simulink model "robotarm_part_2"  (R2018b)
settings: Solver=FixedStepAuto  StartTime=0.0  StopTime=options.T_train  RelTol=1e-3  AbsTol=1e-6
undefined symbols (not defined in the file): options
libraries: neural x132, simulink x2
(part 2 of 6)

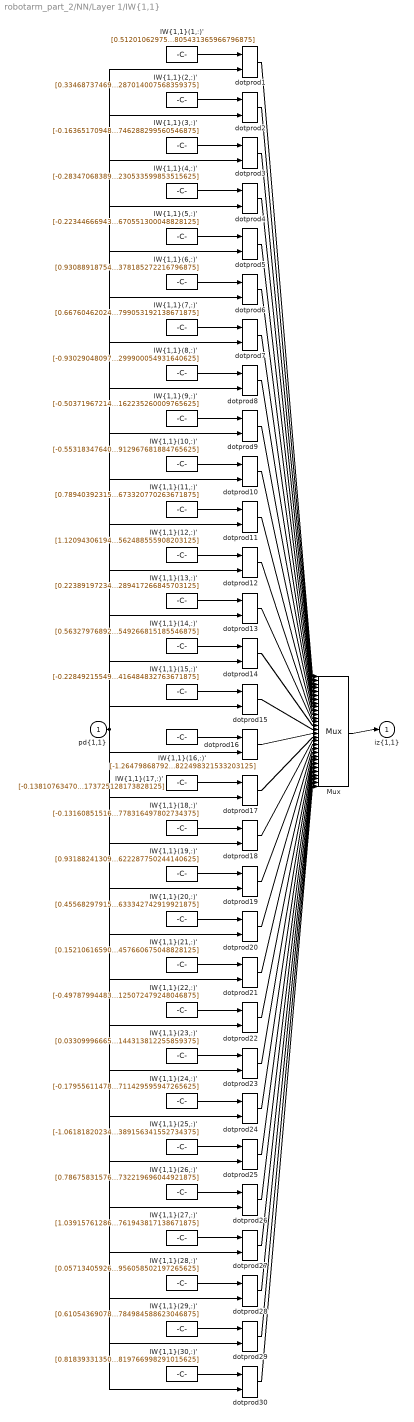
== system robotarm_part_2/NN/Layer 1/IW{1,1} ==
  "pd{1,1}" : Inport  PortDimensions=10
      mask Display: e = 0.06;c1 = [120 230 180]/255;c2 = ([120 230 180]+0)/(256+128);c3 = ([120 230 180]+128)/(256+128);patch([0 1 1 0],[0 0 1 1],c1);patch([0 1 1 1-e 1-e 0+e],[0 0 1 1-e 0+e 0+e],c2);patch([0 0 1 1-e 0+e 0+e],[0 1 1 1-e 1-e 0+e],c3);plot([0 1 1 0 0],[0 0 1 1 0]);
  "IW{1,1}(1,:)'" : Constant  Value=[0.51201062975041689018240731456899084150791168212890625;-0.446218385660316740892739062473992817103862762451171875;-0.82313455567312721061767888386384584009647369384765625;0.67500458565279519707047484189388342201709747314453125;-1.0822077647345456075100855741766281425952911376953125;0.744755827537209480482260914868675172328948974609375;0.61245740151635452708234197416459210216999053955078125;-0.411857215597841774812337689581909216940402984619140625;-0.060313846036639418013436397814075462520122528076171875;0.149541145773167016841398435644805431365966796875]
      mask Display: e = 0.06;c1 = [120 150 230]/255;c2 = ([120 150 230]+0)/383;c3 = ([120 150 230]+128)/383;patch([0 1 1 0],[0 0 1 1],c1);patch([0 1 1 1-e 1-e 0+e],[0 0 1 1-e 0+e 0+e],c2);patch([0 0 1 1-e 0+e 0+e],[0 1 1 1-e 1-e 0+e],c3);plot([0 1 1 0 0],[0 0 1 1 0]);disp('Weights');
  "IW{1,1}(10,:)'" : Constant  Value=[-0.5531834764078296107214782750816084444522857666015625;0.84193722423272554511441967406426556408405303955078125;-0.2314244047025942052631108936111559160053730010986328125;1.268304889703578464121846991474740207195281982421875;-0.298486853726749934434536726257647387683391571044921875;-0.58903786713781192130312547305948100984096527099609375;-0.144387121841211774064817063845111988484859466552734375;1.0323527503820091322239704823005013167858123779296875;-0.5268015142183148924459601403214037418365478515625;-0.294966032842409353609269828666583634912967681884765625]
      mask Display: e = 0.06;c1 = [120 150 230]/255;c2 = ([120 150 230]+0)/383;c3 = ([120 150 230]+128)/383;patch([0 1 1 0],[0 0 1 1],c1);patch([0 1 1 1-e 1-e 0+e],[0 0 1 1-e 0+e 0+e],c2);patch([0 0 1 1-e 0+e 0+e],[0 1 1 1-e 1-e 0+e],c3);plot([0 1 1 0 0],[0 0 1 1 0]);disp('Weights');
  "IW{1,1}(11,:)'" : Constant  Value=[0.78940392315049578986219103171606548130512237548828125;-0.59945395218989439012347020252491347491741180419921875;0.301682263197468436555226389828021638095378875732421875;0.250976303480782869659293510267161764204502105712890625;-0.270480787649907572500751484767533838748931884765625;-0.804027705366989753343887059600092470645904541015625;1.2521368901740081991391662086243741214275360107421875;0.657348093834792646106279789819382131099700927734375;-0.146075233696211059797320785946794785559177398681640625;-0.1885013219685194030272867848907480947673320770263671875]
      mask Display: e = 0.06;c1 = [120 150 230]/255;c2 = ([120 150 230]+0)/383;c3 = ([120 150 230]+128)/383;patch([0 1 1 0],[0 0 1 1],c1);patch([0 1 1 1-e 1-e 0+e],[0 0 1 1-e 0+e 0+e],c2);patch([0 0 1 1-e 0+e 0+e],[0 1 1 1-e 1-e 0+e],c3);plot([0 1 1 0 0],[0 0 1 1 0]);disp('Weights');
  "IW{1,1}(12,:)'" : Constant  Value=[1.120943061943604934782570126117207109928131103515625;-0.1777527950664744837983022307525970973074436187744140625;1.1402714559446653908025837154127657413482666015625;1.6329959194421557189258464859449304640293121337890625;1.799945318979037978124324581585824489593505859375;0.8358067878004415973691720864735543727874755859375;1.064775855755599298646529859979636967182159423828125;-0.152682851516850404127723095371038652956485748291015625;-0.96941769778080966180056066150427795946598052978515625;-0.644809351839978450726675873738713562488555908203125]
      mask Display: e = 0.06;c1 = [120 150 230]/255;c2 = ([120 150 230]+0)/383;c3 = ([120 150 230]+128)/383;patch([0 1 1 0],[0 0 1 1],c1);patch([0 1 1 1-e 1-e 0+e],[0 0 1 1-e 0+e 0+e],c2);patch([0 0 1 1-e 0+e 0+e],[0 1 1 1-e 1-e 0+e],c3);plot([0 1 1 0 0],[0 0 1 1 0]);disp('Weights');
  "IW{1,1}(13,:)'" : Constant  Value=[0.2238919723487180213350455915133352391421794891357421875;0.597710842623245586224811631836928427219390869140625;-0.055930922318855595676279079953019390814006328582763671875;0.97815912828886653063165113053401000797748565673828125;-0.5914319335257880450029688290669582784175872802734375;-0.595428981931443335184894749545492231845855712890625;0.0681264786780833853097050223368569277226924896240234375;1.1822948963348218764934927094145677983760833740234375;0.014091328986622152219521098004406667314469814300537109375;-0.232872425589578935234413847865653224289417266845703125]
      mask Display: e = 0.06;c1 = [120 150 230]/255;c2 = ([120 150 230]+0)/383;c3 = ([120 150 230]+128)/383;patch([0 1 1 0],[0 0 1 1],c1);patch([0 1 1 1-e 1-e 0+e],[0 0 1 1-e 0+e 0+e],c2);patch([0 0 1 1-e 0+e 0+e],[0 1 1 1-e 1-e 0+e],c3);plot([0 1 1 0 0],[0 0 1 1 0]);disp('Weights');
  "IW{1,1}(14,:)'" : Constant  Value=[0.56327976892860409652286080017802305519580841064453125;-0.83851149677898872969450394521118141710758209228515625;0.3782787095400166332836988658527843654155731201171875;-0.2423293037754235268455005325449747033417224884033203125;-0.60723210282409489924049239562009461224079132080078125;1.3496313158650192765009023787570185959339141845703125;-1.068818057232499452169349751784466207027435302734375;0.428137373095577367099195953414891846477985382080078125;0.70485126250453256080419350837473757565021514892578125;-0.304558790502350074103077304243925027549266815185546875]
      mask Display: e = 0.06;c1 = [120 150 230]/255;c2 = ([120 150 230]+0)/383;c3 = ([120 150 230]+128)/383;patch([0 1 1 0],[0 0 1 1],c1);patch([0 1 1 1-e 1-e 0+e],[0 0 1 1-e 0+e 0+e],c2);patch([0 0 1 1-e 0+e 0+e],[0 1 1 1-e 1-e 0+e],c3);plot([0 1 1 0 0],[0 0 1 1 0]);disp('Weights');
  "IW{1,1}(15,:)'" : Constant  Value=[-0.2284921554935588627888165547119569964706897735595703125;1.3167348428603504739697882541804574429988861083984375;-1.183745976367202690227031780523248016834259033203125;0.3104414845865590688589463752578012645244598388671875;-0.24879563196083387399681896567926742136478424072265625;-0.8014990752859769695959357704850845038890838623046875;0.97682041688133935952720321438391692936420440673828125;0.9148661125020822737496928311884403228759765625;-0.53839922957077013254689745735959149897098541259765625;0.0629641058630556471609196478311787359416484832763671875]
      mask Display: e = 0.06;c1 = [120 150 230]/255;c2 = ([120 150 230]+0)/383;c3 = ([120 150 230]+128)/383;patch([0 1 1 0],[0 0 1 1],c1);patch([0 1 1 1-e 1-e 0+e],[0 0 1 1-e 0+e 0+e],c2);patch([0 0 1 1-e 0+e 0+e],[0 1 1 1-e 1-e 0+e],c3);plot([0 1 1 0 0],[0 0 1 1 0]);disp('Weights');
  "IW{1,1}(16,:)'" : Constant  Value=[-1.264798687929534093399297489668242633342742919921875;-0.8666288950522902378992284866399131715297698974609375;-0.351867621039619382639074274266022257506847381591796875;-1.2235468539213540939414315289468504488468170166015625;-0.69647725102835267296796928349067457020282745361328125;-0.336143791072206876702210820440086536109447479248046875;-2.07998144178045407670651911757886409759521484375;0.42152524350633291394530033358023501932621002197265625;-0.54013888040281232694184154752292670309543609619140625;0.27962398287528611451335791571182198822498321533203125]
      mask Display: e = 0.06;c1 = [120 150 230]/255;c2 = ([120 150 230]+0)/383;c3 = ([120 150 230]+128)/383;patch([0 1 1 0],[0 0 1 1],c1);patch([0 1 1 1-e 1-e 0+e],[0 0 1 1-e 0+e 0+e],c2);patch([0 0 1 1-e 0+e 0+e],[0 1 1 1-e 1-e 0+e],c3);plot([0 1 1 0 0],[0 0 1 1 0]);disp('Weights');
  "IW{1,1}(17,:)'" : Constant  Value=[-0.138107634700562698082393353615771047770977020263671875;-0.6829199452269809622606544508016668260097503662109375;0.1872812962193503294461294217398972250521183013916015625;0.996618728469853554230439840466715395450592041015625;0.70601568915720169794525418183184228837490081787109375;0.71409007827887716057801981150987558066844940185546875;-0.05393398252795689185035143964341841638088226318359375;0.54491065742438049568363567232154309749603271484375;0.71411317961737508230868343162001110613346099853515625;-0.1686958312051092534478158313504536636173725128173828125]
      mask Display: e = 0.06;c1 = [120 150 230]/255;c2 = ([120 150 230]+0)/383;c3 = ([120 150 230]+128)/383;patch([0 1 1 0],[0 0 1 1],c1);patch([0 1 1 1-e 1-e 0+e],[0 0 1 1-e 0+e 0+e],c2);patch([0 0 1 1-e 0+e 0+e],[0 1 1 1-e 1-e 0+e],c3);plot([0 1 1 0 0],[0 0 1 1 0]);disp('Weights');
  "IW{1,1}(18,:)'" : Constant  Value=[-0.1316085151623478111115872479786048643290996551513671875;0.1705613878097677893475037080861511640250682830810546875;-0.0962470582835133203758459785603918135166168212890625;-0.91249714780919777279422078208881430327892303466796875;-1.158643775472975701035238671465776860713958740234375;0.068576612657344160339789596037007868289947509765625;0.35933323325870480946520046927616931498050689697265625;0.93664609339309568003528738699969835579395294189453125;0.6175964938953411031974383149645291268825531005859375;0.53882994034340947475669736377312801778316497802734375]
      mask Display: e = 0.06;c1 = [120 150 230]/255;c2 = ([120 150 230]+0)/383;c3 = ([120 150 230]+128)/383;patch([0 1 1 0],[0 0 1 1],c1);patch([0 1 1 1-e 1-e 0+e],[0 0 1 1-e 0+e 0+e],c2);patch([0 0 1 1-e 0+e 0+e],[0 1 1 1-e 1-e 0+e],c3);plot([0 1 1 0 0],[0 0 1 1 0]);disp('Weights');
  "IW{1,1}(19,:)'" : Constant  Value=[0.93188241309977526416474802317679859697818756103515625;0.3431987483161054175440085600712336599826812744140625;0.8149782526990210218542642905958928167819976806640625;-0.48223366783551668834917336425860412418842315673828125;-1.2205060054262257818180614776792936027050018310546875;-0.518485301399788767184872995130717754364013671875;0.1822236035677796961440577661051065661013126373291015625;0.59438057885021955417670369570259936153888702392578125;0.290405258873669025465602544500143267214298248291015625;-0.227514175994425971172319123070337809622287750244140625]
      mask Display: e = 0.06;c1 = [120 150 230]/255;c2 = ([120 150 230]+0)/383;c3 = ([120 150 230]+128)/383;patch([0 1 1 0],[0 0 1 1],c1);patch([0 1 1 1-e 1-e 0+e],[0 0 1 1-e 0+e 0+e],c2);patch([0 0 1 1-e 0+e 0+e],[0 1 1 1-e 1-e 0+e],c3);plot([0 1 1 0 0],[0 0 1 1 0]);disp('Weights');
  "IW{1,1}(2,:)'" : Constant  Value=[0.334687374696120254480291578147443942725658416748046875;0.8542580739553733426561166197643615305423736572265625;-0.300144445451211716591188860547845251858234405517578125;0.208731003203754206243303315204684622585773468017578125;-0.85850869408691499184982376391417346894741058349609375;-0.8662264510329513722552974286372773349285125732421875;0.22452379060819982470320610445924103260040283203125;0.15532066551018408606665843763039447367191314697265625;0.1101313638464642696845885438960976898670196533203125;-0.869876084554048301100692697218619287014007568359375]
      mask Display: e = 0.06;c1 = [120 150 230]/255;c2 = ([120 150 230]+0)/383;c3 = ([120 150 230]+128)/383;patch([0 1 1 0],[0 0 1 1],c1);patch([0 1 1 1-e 1-e 0+e],[0 0 1 1-e 0+e 0+e],c2);patch([0 0 1 1-e 0+e 0+e],[0 1 1 1-e 1-e 0+e],c3);plot([0 1 1 0 0],[0 0 1 1 0]);disp('Weights');
  "IW{1,1}(20,:)'" : Constant  Value=[0.455682979150963729519929756861529313027858734130859375;-0.348772677236663664057658706951770000159740447998046875;-1.081291878654035532036914446507580578327178955078125;0.6215181655236268198905236204154789447784423828125;-1.26078388760682447156113994424231350421905517578125;0.26210421145090878614070106777944602072238922119140625;-0.8124006863890798069149923321674577891826629638671875;-0.7488565667669575542930715528200380504131317138671875;-0.022788057892801479031863465252172318287193775177001953125;-0.569162418060251251716863407636992633342742919921875]
      mask Display: e = 0.06;c1 = [120 150 230]/255;c2 = ([120 150 230]+0)/383;c3 = ([120 150 230]+128)/383;patch([0 1 1 0],[0 0 1 1],c1);patch([0 1 1 1-e 1-e 0+e],[0 0 1 1-e 0+e 0+e],c2);patch([0 0 1 1-e 0+e 0+e],[0 1 1 1-e 1-e 0+e],c3);plot([0 1 1 0 0],[0 0 1 1 0]);disp('Weights');
  "IW{1,1}(21,:)'" : Constant  Value=[0.15210616590676995230069223907776176929473876953125;-0.52353059267904367146684307954274117946624755859375;-0.06401275842094468482290636757170432247221469879150390625;0.8786379509407431509515618017758242785930633544921875;-0.984808213135992094322546108742244541645050048828125;-0.80881132688778212269653522525914013385772705078125;1.0254205955323396626255316732567735016345977783203125;-0.572903581729212962869723924086429178714752197265625;-0.57828165266377162812005963132833130657672882080078125;-0.0981817788360586363172188839598675258457660675048828125]
      mask Display: e = 0.06;c1 = [120 150 230]/255;c2 = ([120 150 230]+0)/383;c3 = ([120 150 230]+128)/383;patch([0 1 1 0],[0 0 1 1],c1);patch([0 1 1 1-e 1-e 0+e],[0 0 1 1-e 0+e 0+e],c2);patch([0 0 1 1-e 0+e 0+e],[0 1 1 1-e 1-e 0+e],c3);plot([0 1 1 0 0],[0 0 1 1 0]);disp('Weights');
  "IW{1,1}(22,:)'" : Constant  Value=[-0.49787994483490027874950101249851286411285400390625;0.344426173820214842624665152470697648823261260986328125;0.56655019007916529449886411384795792400836944580078125;-0.1743990939602932666030454811334493570029735565185546875;-0.55634090371249012019205792967113666236400604248046875;0.89898279581140183580600933055393397808074951171875;-0.879074509234978318517050865921191871166229248046875;0.35855501727174743376025389807182364165782928466796875;-0.35938092675222998995110401665442623198032379150390625;0.259808285173537878431915260080131702125072479248046875]
      mask Display: e = 0.06;c1 = [120 150 230]/255;c2 = ([120 150 230]+0)/383;c3 = ([120 150 230]+128)/383;patch([0 1 1 0],[0 0 1 1],c1);patch([0 1 1 1-e 1-e 0+e],[0 0 1 1-e 0+e 0+e],c2);patch([0 0 1 1-e 0+e 0+e],[0 1 1 1-e 1-e 0+e],c3);plot([0 1 1 0 0],[0 0 1 1 0]);disp('Weights');
  "IW{1,1}(23,:)'" : Constant  Value=[0.033099966659816792979853516953880898654460906982421875;0.06638646623711309813220537989764125086367130279541015625;-0.68962437461610448519166993719409219920635223388671875;-0.7036292898254934424784323709900490939617156982421875;1.2199498264654824453145920415408909320831298828125;-0.79167659947821267252265897695906460285186767578125;-0.77727190827501690950640522714820690453052520751953125;-0.86932059827218122194381066947244107723236083984375;-1.30799569035398377536694169975817203521728515625;0.61475854294593756943498874534270726144313812255859375]
      mask Display: e = 0.06;c1 = [120 150 230]/255;c2 = ([120 150 230]+0)/383;c3 = ([120 150 230]+128)/383;patch([0 1 1 0],[0 0 1 1],c1);patch([0 1 1 1-e 1-e 0+e],[0 0 1 1-e 0+e 0+e],c2);patch([0 0 1 1-e 0+e 0+e],[0 1 1 1-e 1-e 0+e],c3);plot([0 1 1 0 0],[0 0 1 1 0]);disp('Weights');
  "IW{1,1}(24,:)'" : Constant  Value=[-0.179556114788564202822129800551920197904109954833984375;-1.087956549232024006101937629864551126956939697265625;-0.491519599031757403739817391397082246840000152587890625;0.431654739378498575330667108573834411799907684326171875;-0.5203235292342416329347543069161474704742431640625;1.0774856436627977540609890638734214007854461669921875;-0.78412901417916491819681823471910320222377777099609375;-0.45999524609127895313775979957426898181438446044921875;-0.65676880719675245767774640626157633960247039794921875;-0.044675480221918285883564436744563863612711429595947265625]
      mask Display: e = 0.06;c1 = [120 150 230]/255;c2 = ([120 150 230]+0)/383;c3 = ([120 150 230]+128)/383;patch([0 1 1 0],[0 0 1 1],c1);patch([0 1 1 1-e 1-e 0+e],[0 0 1 1-e 0+e 0+e],c2);patch([0 0 1 1-e 0+e 0+e],[0 1 1 1-e 1-e 0+e],c3);plot([0 1 1 0 0],[0 0 1 1 0]);disp('Weights');
  "IW{1,1}(25,:)'" : Constant  Value=[-1.0618182023466058438998516066931188106536865234375;0.79817916296788327112921024308889172971248626708984375;0.66539862575941655098432647719164378941059112548828125;-0.051018015239275439631772002258003340102732181549072265625;-1.0134808839080953202227419751579873263835906982421875;0.32366586780373907128449673109571449458599090576171875;-0.77640544809128508862983153449022211134433746337890625;0.052087738911195731461578617427221615798771381378173828125;0.356415790452184799708135187756852246820926666259765625;-0.82901405933345040377702162004425190389156341552734375]
      mask Display: e = 0.06;c1 = [120 150 230]/255;c2 = ([120 150 230]+0)/383;c3 = ([120 150 230]+128)/383;patch([0 1 1 0],[0 0 1 1],c1);patch([0 1 1 1-e 1-e 0+e],[0 0 1 1-e 0+e 0+e],c2);patch([0 0 1 1-e 0+e 0+e],[0 1 1 1-e 1-e 0+e],c3);plot([0 1 1 0 0],[0 0 1 1 0]);disp('Weights');
  "IW{1,1}(26,:)'" : Constant  Value=[0.7867583157629229884122423754888586699962615966796875;-0.09876131895016322659319740751016070134937763214111328125;0.040937343456810305897253243756495066918432712554931640625;-0.6377087573054336377964546045404858887195587158203125;0.92183111098579606501601801937795244157314300537109375;0.7630701117262292942911017235019244253635406494140625;-0.9559463989704750641607233774266205728054046630859375;0.0083999903600966881189737733848232892341911792755126953125;0.28071027682913085588012336302199400961399078369140625;-0.356962075893640651269578256687964312732219696044921875]
      mask Display: e = 0.06;c1 = [120 150 230]/255;c2 = ([120 150 230]+0)/383;c3 = ([120 150 230]+128)/383;patch([0 1 1 0],[0 0 1 1],c1);patch([0 1 1 1-e 1-e 0+e],[0 0 1 1-e 0+e 0+e],c2);patch([0 0 1 1-e 0+e 0+e],[0 1 1 1-e 1-e 0+e],c3);plot([0 1 1 0 0],[0 0 1 1 0]);disp('Weights');
  "IW{1,1}(27,:)'" : Constant  Value=[1.0391576128606516693508865500916726887226104736328125;-0.68078374226108329114737216514186002314090728759765625;-0.84542657228553519388469794648699462413787841796875;0.182872090681562127212345103544066660106182098388671875;0.201449348403338335256052005206583999097347259521484375;1.2222722009825515154801678363583050668239593505859375;-0.209857643206624533416260192097979597747325897216796875;-0.0260964357222159791527271721633951528929173946380615234375;0.032308480457565631749350387735830736346542835235595703125;-0.32241355661655546338550948348711244761943817138671875]
      mask Display: e = 0.06;c1 = [120 150 230]/255;c2 = ([120 150 230]+0)/383;c3 = ([120 150 230]+128)/383;patch([0 1 1 0],[0 0 1 1],c1);patch([0 1 1 1-e 1-e 0+e],[0 0 1 1-e 0+e 0+e],c2);patch([0 0 1 1-e 0+e 0+e],[0 1 1 1-e 1-e 0+e],c3);plot([0 1 1 0 0],[0 0 1 1 0]);disp('Weights');
  "IW{1,1}(28,:)'" : Constant  Value=[0.057134059266083149497550408568713464774191379547119140625;0.9612957029473683245868187441374175250530242919921875;-0.82745424130805333984284288817434571683406829833984375;-0.358522123753254928768541276440373621881008148193359375;-0.370650427652782610277171215784619562327861785888671875;0.79355103244975133680583212480996735394001007080078125;-0.585900745193040695113495530677028000354766845703125;-0.3012560077043449080491654967772774398326873779296875;-0.59586095918726922349151209346018731594085693359375;0.06521372026171236291336441581734106875956058502197265625]
      mask Display: e = 0.06;c1 = [120 150 230]/255;c2 = ([120 150 230]+0)/383;c3 = ([120 150 230]+128)/383;patch([0 1 1 0],[0 0 1 1],c1);patch([0 1 1 1-e 1-e 0+e],[0 0 1 1-e 0+e 0+e],c2);patch([0 0 1 1-e 0+e 0+e],[0 1 1 1-e 1-e 0+e],c3);plot([0 1 1 0 0],[0 0 1 1 0]);disp('Weights');
  "IW{1,1}(29,:)'" : Constant  Value=[0.61054369078136849768867477905587293207645416259765625;0.285441813611004846507057663984596729278564453125;0.82694574023073530444349898971267975866794586181640625;-0.95255589439435184306859127900679595768451690673828125;-0.7232895052037340288819677880383096635341644287109375;0.052786005032112760793072681053672567941248416900634765625;0.32963064971604894015655418115784414112567901611328125;-0.361308139964405972133221212061471305787563323974609375;-0.0607358777905373237171460232275421731173992156982421875;0.365889917645603357509997977103921584784984588623046875]
      mask Display: e = 0.06;c1 = [120 150 230]/255;c2 = ([120 150 230]+0)/383;c3 = ([120 150 230]+128)/383;patch([0 1 1 0],[0 0 1 1],c1);patch([0 1 1 1-e 1-e 0+e],[0 0 1 1-e 0+e 0+e],c2);patch([0 0 1 1-e 0+e 0+e],[0 1 1 1-e 1-e 0+e],c3);plot([0 1 1 0 0],[0 0 1 1 0]);disp('Weights');
  "IW{1,1}(3,:)'" : Constant  Value=[-0.1636517094816495043740900428019813261926174163818359375;0.2790709887831928082135846125311218202114105224609375;-0.82095080725694657974855772408773191273212432861328125;0.90315988282876080717187505797483026981353759765625;-0.585383166098789597953100383165292441844940185546875;-0.9028020381220780432585115704569034278392791748046875;-0.55194084143176491696891616811626590788364410400390625;-0.80841281361235195479508774951682426035404205322265625;-0.1330243909813022262778048343534464947879314422607421875;-0.79353581713547594045365940473857335746288299560546875]
      mask Display: e = 0.06;c1 = [120 150 230]/255;c2 = ([120 150 230]+0)/383;c3 = ([120 150 230]+128)/383;patch([0 1 1 0],[0 0 1 1],c1);patch([0 1 1 1-e 1-e 0+e],[0 0 1 1-e 0+e 0+e],c2);patch([0 0 1 1-e 0+e 0+e],[0 1 1 1-e 1-e 0+e],c3);plot([0 1 1 0 0],[0 0 1 1 0]);disp('Weights');
  "IW{1,1}(30,:)'" : Constant  Value=[0.81839331350390442931796997072524391114711761474609375;-0.65665848396522774610417627627612091600894927978515625;-0.62904998603653716759964709126506932079792022705078125;-0.244816186549569547725724305564654059708118438720703125;0.7943841339580812732634740314097143709659576416015625;0.9540530841623862112754750341991893947124481201171875;0.222742363091552320053523317255894653499126434326171875;-0.40821844777976334928126789236557669937610626220703125;-0.5056520505561186151766150942421518266201019287109375;0.5224344282092714397691679550916887819766998291015625]
      mask Display: e = 0.06;c1 = [120 150 230]/255;c2 = ([120 150 230]+0)/383;c3 = ([120 150 230]+128)/383;patch([0 1 1 0],[0 0 1 1],c1);patch([0 1 1 1-e 1-e 0+e],[0 0 1 1-e 0+e 0+e],c2);patch([0 0 1 1-e 0+e 0+e],[0 1 1 1-e 1-e 0+e],c3);plot([0 1 1 0 0],[0 0 1 1 0]);disp('Weights');
  "IW{1,1}(4,:)'" : Constant  Value=[-0.283470683898927433563841304930974729359149932861328125;-0.566705526229471789889657884486950933933258056640625;-0.0683239219797149299751026774174533784389495849609375;-0.334143830811465314400976467368309386074542999267578125;-0.7385101067126182972089054601383395493030548095703125;0.085369537996802635770876577225863002240657806396484375;0.508384686137323793531095361686311662197113037109375;1.3096152971670582676466665361658670008182525634765625;-0.80825421096264238318696015994646586477756500244140625;-0.73138548990404628202810499715269543230533599853515625]
      mask Display: e = 0.06;c1 = [120 150 230]/255;c2 = ([120 150 230]+0)/383;c3 = ([120 150 230]+128)/383;patch([0 1 1 0],[0 0 1 1],c1);patch([0 1 1 1-e 1-e 0+e],[0 0 1 1-e 0+e 0+e],c2);patch([0 0 1 1-e 0+e 0+e],[0 1 1 1-e 1-e 0+e],c3);plot([0 1 1 0 0],[0 0 1 1 0]);disp('Weights');
  "IW{1,1}(5,:)'" : Constant  Value=[-0.22344666943307378570438004317111335694789886474609375;0.55446481881344722442150896313250996172428131103515625;-0.6986360943472436080270426828064955770969390869140625;0.1859580900224321042824016103622852824628353118896484375;-0.67870494890880450622461239618132822215557098388671875;-0.586692796095814816936808711034245789051055908203125;0.09071355422038583637966979722477844916284084320068359375;0.25741529128786100333314834642806090414524078369140625;-0.77523298959876674185665024197078309953212738037109375;-0.3024283743969693460940106888301670551300048828125]
      mask Display: e = 0.06;c1 = [120 150 230]/255;c2 = ([120 150 230]+0)/383;c3 = ([120 150 230]+128)/383;patch([0 1 1 0],[0 0 1 1],c1);patch([0 1 1 1-e 1-e 0+e],[0 0 1 1-e 0+e 0+e],c2);patch([0 0 1 1-e 0+e 0+e],[0 1 1 1-e 1-e 0+e],c3);plot([0 1 1 0 0],[0 0 1 1 0]);disp('Weights');
  "IW{1,1}(6,:)'" : Constant  Value=[0.9308891875477172117570034970412962138652801513671875;0.6248987167310067203374046584940515458583831787109375;-0.421406323878703081842189703820622526109218597412109375;-0.5088996357030708406199437376926653087139129638671875;-0.8857877018437314564636153590981848537921905517578125;-0.2069905306570896386109126297014881856739521026611328125;-1.0089923907319573448404526061494834721088409423828125;0.08415741437822508996813297699191025458276271820068359375;0.97591180294049617582885502997669391334056854248046875;-0.388183431962278557847412230330519378185272216796875]
      mask Display: e = 0.06;c1 = [120 150 230]/255;c2 = ([120 150 230]+0)/383;c3 = ([120 150 230]+128)/383;patch([0 1 1 0],[0 0 1 1],c1);patch([0 1 1 1-e 1-e 0+e],[0 0 1 1-e 0+e 0+e],c2);patch([0 0 1 1-e 0+e 0+e],[0 1 1 1-e 1-e 0+e],c3);plot([0 1 1 0 0],[0 0 1 1 0]);disp('Weights');
  "IW{1,1}(7,:)'" : Constant  Value=[0.66760462024022715343818390465457923710346221923828125;-0.333285831523196518499929652534774504601955413818359375;0.0154658587186106109834238253597504808567464351654052734375;0.015814647545966863118049872127812705002725124359130859375;-0.81793240186973459326935653734835796058177947998046875;-0.33959407024115029205546534285531379282474517822265625;-1.5662660277990558821414879275835119187831878662109375;-0.87198956266450411423107880182215012609958648681640625;0.351466567986612410390279137573088519275188446044921875;0.398619991678556828684776291993330232799053192138671875]
      mask Display: e = 0.06;c1 = [120 150 230]/255;c2 = ([120 150 230]+0)/383;c3 = ([120 150 230]+128)/383;patch([0 1 1 0],[0 0 1 1],c1);patch([0 1 1 1-e 1-e 0+e],[0 0 1 1-e 0+e 0+e],c2);patch([0 0 1 1-e 0+e 0+e],[0 1 1 1-e 1-e 0+e],c3);plot([0 1 1 0 0],[0 0 1 1 0]);disp('Weights');
  "IW{1,1}(8,:)'" : Constant  Value=[-0.9302904809764058757792781761963851749897003173828125;0.45922692721911317903504823334515094757080078125;-0.95093316525850790643659138368093408644199371337890625;-0.93733031649115894357038314410601742565631866455078125;-0.10339789326997579632649859604498487897217273712158203125;0.476935800121459585465544250837410800158977508544921875;0.47368795097230564916657158391899429261684417724609375;0.149512630423817183267232167054316960275173187255859375;-0.87451657742440003229233980164281092584133148193359375;-0.06311678743072259012425462287865229882299900054931640625]
      mask Display: e = 0.06;c1 = [120 150 230]/255;c2 = ([120 150 230]+0)/383;c3 = ([120 150 230]+128)/383;patch([0 1 1 0],[0 0 1 1],c1);patch([0 1 1 1-e 1-e 0+e],[0 0 1 1-e 0+e 0+e],c2);patch([0 0 1 1-e 0+e 0+e],[0 1 1 1-e 1-e 0+e],c3);plot([0 1 1 0 0],[0 0 1 1 0]);disp('Weights');
  "IW{1,1}(9,:)'" : Constant  Value=[-0.50371967214158874792673259435105137526988983154296875;0.952248675876548933416643194505013525485992431640625;0.1863763124311817731548757137716165743768215179443359375;-0.5063200098583349184622193206450901925563812255859375;0.50613566425012901373037266239407472312450408935546875;-0.398276942527581445663287240677163936197757720947265625;1.141547367716243766011530169635079801082611083984375;-0.1390199499433947549764667428462416864931583404541015625;-0.30553120975796244085387343147885985672473907470703125;-0.16884738415671896039071953055099584162235260009765625]
      mask Display: e = 0.06;c1 = [120 150 230]/255;c2 = ([120 150 230]+0)/383;c3 = ([120 150 230]+128)/383;patch([0 1 1 0],[0 0 1 1],c1);patch([0 1 1 1-e 1-e 0+e],[0 0 1 1-e 0+e 0+e],c2);patch([0 0 1 1-e 0+e 0+e],[0 1 1 1-e 1-e 0+e],c3);plot([0 1 1 0 0],[0 0 1 1 0]);disp('Weights');
  Mux : Mux  Inputs=30
      mask Display: e = 0.06;c1 = [120 150 230]/255;c2 = ([120 150 230]+0)/383;c3 = ([120 150 230]+128)/383;patch([0 1 1 0],[0 0 1 1],c1);patch([0 1 1 1-e 1-e 0+e],[0 0 1 1-e 0+e 0+e],c2);patch([0 0 1 1-e 0+e 0+e],[0 1 1 1-e 1-e 0+e],c3);plot([0 1 1 0 0],[0 0 1 1 0]);disp('Mux');
  dotprod{1..30} (30 alike) : neural/Weight Functions/dotprod
  "iz{1,1}" : Outport
      mask Display: e = 0.06;c1 = [120 230 180]/255;c2 = ([120 230 180]+0)/(256+128);c3 = ([120 230 180]+128)/(256+128);patch([0 1 1 0],[0 0 1 1],c1);patch([0 1 1 1-e 1-e 0+e],[0 0 1 1-e 0+e 0+e],c2);patch([0 0 1 1-e 0+e 0+e],[0 1 1 1-e 1-e 0+e],c3);plot([0 1 1 0 0],[0 0 1 1 0]);
  wires:
  "IW{1,1}(1,:)'"/1 -> dotprod1/1
  "pd{1,1}"/1 -> dotprod1/2, dotprod2/2, dotprod3/2, dotprod4/2, dotprod5/2, dotprod6/2, dotprod7/2, dotprod8/2, dotprod9/2, dotprod10/2, dotprod11/2, dotprod12/2, dotprod13/2, dotprod14/2, dotprod15/2, dotprod16/2, dotprod17/2, dotprod18/2, dotprod19/2, dotprod20/2, dotprod21/2, dotprod22/2, dotprod23/2, dotprod24/2, dotprod25/2, dotprod26/2, dotprod27/2, dotprod28/2, dotprod29/2, dotprod30/2
  dotprod1/1 -> Mux/1
  "IW{1,1}(2,:)'"/1 -> dotprod2/1
  dotprod2/1 -> Mux/2
  "IW{1,1}(3,:)'"/1 -> dotprod3/1
  dotprod3/1 -> Mux/3
  "IW{1,1}(4,:)'"/1 -> dotprod4/1
  dotprod4/1 -> Mux/4
  "IW{1,1}(5,:)'"/1 -> dotprod5/1
  dotprod5/1 -> Mux/5
  "IW{1,1}(6,:)'"/1 -> dotprod6/1
  dotprod6/1 -> Mux/6
  "IW{1,1}(7,:)'"/1 -> dotprod7/1
  dotprod7/1 -> Mux/7
  "IW{1,1}(8,:)'"/1 -> dotprod8/1
  dotprod8/1 -> Mux/8
  "IW{1,1}(9,:)'"/1 -> dotprod9/1
  dotprod9/1 -> Mux/9
  "IW{1,1}(10,:)'"/1 -> dotprod10/1
  dotprod10/1 -> Mux/10
  "IW{1,1}(11,:)'"/1 -> dotprod11/1
  dotprod11/1 -> Mux/11
  "IW{1,1}(12,:)'"/1 -> dotprod12/1
  dotprod12/1 -> Mux/12
  "IW{1,1}(13,:)'"/1 -> dotprod13/1
  dotprod13/1 -> Mux/13
  "IW{1,1}(14,:)'"/1 -> dotprod14/1
  dotprod14/1 -> Mux/14
  "IW{1,1}(15,:)'"/1 -> dotprod15/1
  dotprod15/1 -> Mux/15
  "IW{1,1}(16,:)'"/1 -> dotprod16/1
  dotprod16/1 -> Mux/16
  "IW{1,1}(17,:)'"/1 -> dotprod17/1
  dotprod17/1 -> Mux/17
  "IW{1,1}(18,:)'"/1 -> dotprod18/1
  dotprod18/1 -> Mux/18
  "IW{1,1}(19,:)'"/1 -> dotprod19/1
  dotprod19/1 -> Mux/19
  "IW{1,1}(20,:)'"/1 -> dotprod20/1
  dotprod20/1 -> Mux/20
  "IW{1,1}(21,:)'"/1 -> dotprod21/1
  dotprod21/1 -> Mux/21
  "IW{1,1}(22,:)'"/1 -> dotprod22/1
  dotprod22/1 -> Mux/22
  "IW{1,1}(23,:)'"/1 -> dotprod23/1
  dotprod23/1 -> Mux/23
  "IW{1,1}(24,:)'"/1 -> dotprod24/1
  dotprod24/1 -> Mux/24
  "IW{1,1}(25,:)'"/1 -> dotprod25/1
  dotprod25/1 -> Mux/25
  "IW{1,1}(26,:)'"/1 -> dotprod26/1
  dotprod26/1 -> Mux/26
  "IW{1,1}(27,:)'"/1 -> dotprod27/1
  dotprod27/1 -> Mux/27
  "IW{1,1}(28,:)'"/1 -> dotprod28/1
  dotprod28/1 -> Mux/28
  "IW{1,1}(29,:)'"/1 -> dotprod29/1
  dotprod29/1 -> Mux/29
  "IW{1,1}(30,:)'"/1 -> dotprod30/1
  dotprod30/1 -> Mux/30
  Mux/1 -> "iz{1,1}"/1

== system robotarm_part_2/NN/Layer 2/Delays 1 ==
  "p{2}" : Inport  PortDimensions=30
      mask Display: e = 0.06;c1 = [120 230 180]/255;c2 = ([120 230 180]+0)/(256+128);c3 = ([120 230 180]+128)/(256+128);patch([0 1 1 0],[0 0 1 1],c1);patch([0 1 1 1-e 1-e 0+e],[0 0 1 1-e 0+e 0+e],c2);patch([0 0 1 1-e 0+e 0+e],[0 1 1 1-e 1-e 0+e],c3);plot([0 1 1 0 0],[0 0 1 1 0]);
  mux : Mux  Inputs=1
      mask Display: e = 0.06;c1 = [120 150 230]/255;c2 = ([120 150 230]+0)/383;c3 = ([120 150 230]+128)/383;patch([0 1 1 0],[0 0 1 1],c1);patch([0 1 1 1-e 1-e 0+e],[0 0 1 1-e 0+e 0+e],c2);patch([0 0 1 1-e 0+e 0+e],[0 1 1 1-e 1-e 0+e],c3);plot([0 1 1 0 0],[0 0 1 1 0]);disp('Mux')
  "pd{2,1}" : Outport
      mask Display: e = 0.06;c1 = [120 230 180]/255;c2 = ([120 230 180]+0)/(256+128);c3 = ([120 230 180]+128)/(256+128);patch([0 1 1 0],[0 0 1 1],c1);patch([0 1 1 1-e 1-e 0+e],[0 0 1 1-e 0+e 0+e],c2);patch([0 0 1 1-e 0+e 0+e],[0 1 1 1-e 1-e 0+e],c3);plot([0 1 1 0 0],[0 0 1 1 0]);
  wires:
  "p{2}"/1 -> mux/1
  mux/1 -> "pd{2,1}"/1
